simulink model "sim_model"  (R2018b)
settings: Solver=VariableStepAuto  StartTime=0.0  StopTime=tf  FixedStep=1e-6  RelTol=1e-3
values from neighbouring files (symbols this model uses):
  g = 9.81    [Main.m]
  L0 = 0.09    [Main.m]
  m = 10e-2    (= 0.1)    [Main.m]
  R = 60    [Main.m]
  u0 = er    [Main.m]
  x10 = 0.03    [Main.m]
  x20 = v0    (= 0)    [Main.m]
  x30 = I0    [Main.m]
settings Model: Creator=Eduardo  LastModifiedBy=ohara

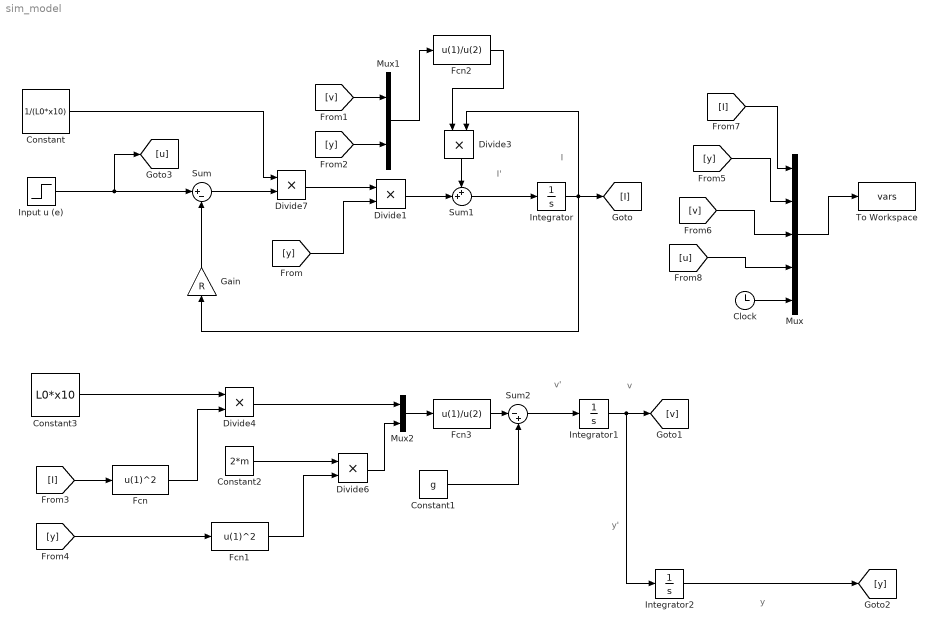
== system sim_model ==
  note: y
  note: y'
  note: v
  note: v'
  note: I'
  note: I
  Clock : Clock
  Constant : Constant  Value=1/(L0*x10)  VectorParams1D=off
  Constant1 : Constant  Value=g
  Constant2 : Constant  Value=2*m
  Constant3 : Constant  Value=L0*x10
  Divide{1,3..4,6..7} (5 alike) : Product  Inputs=**
  Fcn : Fcn  Expr=u(1)^2
  Fcn1 : Fcn  Expr=u(1)^2
  Fcn2 : Fcn  Expr=u(1)/u(2)
  Fcn3 : Fcn  Expr=u(1)/u(2)
  Gain : Gain  Gain=R
  "Input u (e) " : Step  Time=0  Before=u0  After=u0  SampleTime=0
  Integrator : Integrator  InitialCondition=x30
  Integrator1 : Integrator  InitialCondition=x20
  Integrator2 : Integrator  InitialCondition=x10  LimitOutput=on  LowerSaturationLimit=0.001
  Mux : Mux  Inputs=5
  Mux1 : Mux  Inputs=2
  Mux2 : Mux  Inputs=2
  Sum : Sum  Inputs=|+-
  Sum1 : Sum  Inputs=++|
  Sum2 : Sum  Inputs=|-+
  To Workspace : ToWorkspace  VariableName=vars  SaveFormat=Timeseries  SampleTime=-1
  wires:
  Gain/1 -> Sum/2
  Constant/1 -> Divide7/1
  Divide1/1 -> Sum1/2
  Sum1/1 -> Integrator/1
  Integrator/1 -> Gain/1, Divide3/2, [I]
  [y] -> Divide1/2
  Divide3/1 -> Sum1/1
  [I] -> Fcn/1
  Fcn/1 -> Divide4/2
  Constant2/1 -> Divide6/1
  Fcn1/1 -> Divide6/2
  [y] -> Fcn1/1
  Constant1/1 -> Sum2/2
  Sum2/1 -> Integrator1/1
  Integrator1/1 -> Integrator2/1, [v]
  Mux/1 -> To Workspace/1
  [y] -> Mux/2
  [v] -> Mux/3
  [I] -> Mux/1
  Clock/1 -> Mux/5
  [u] -> Mux/4
  Integrator2/1 -> [y]
  "Input u (e) "/1 -> [u], Sum/1
  Divide7/1 -> Divide1/1
  Sum/1 -> Divide7/2
  [y] -> Mux1/2
  [v] -> Mux1/1
  Mux1/1 -> Fcn2/1
  Fcn2/1 -> Divide3/1
  Fcn3/1 -> Sum2/1
  Mux2/1 -> Fcn3/1
  Divide6/1 -> Mux2/2
  Divide4/1 -> Mux2/1
  Constant3/1 -> Divide4/1
